simulink model "RT_ueb3_3a"  (R2013a)
settings: Solver=ode45  StartTime=0.0  StopTime=10.0  RelTol=1e-3
settings Model: BufferReuse=off  Creator=mainster  LastModifiedBy=mainster
settings OptimizationCC: InlineParams=on  BufferReuse=off
settings DebuggingCC: InitInArrayFormatMsg=none

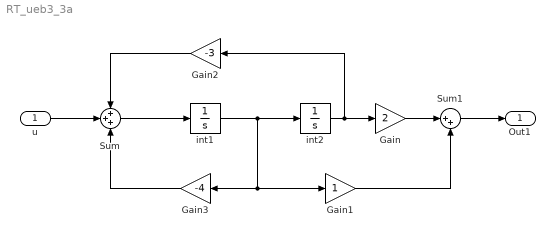
== system RT_ueb3_3a ==
  u : Inport
  Gain : Gain  Gain=2
  Gain1 : Gain
  Gain2 : Gain  Gain=-3
  Gain3 : Gain  Gain=-4
  Sum : Sum  Inputs=+++
  Sum1 : Sum  Inputs=|++
  int1 : Integrator
  int2 : Integrator
  Out1 : Outport
  wires:
  u/1 -> Sum/2
  Sum/1 -> int1/1
  int1/1 -> Gain3/1, Gain1/1, int2/1
  Gain2/1 -> Sum/1
  int2/1 -> Gain/1, Gain2/1
  Gain/1 -> Sum1/1
  Gain1/1 -> Sum1/2
  Sum1/1 -> Out1/1
  Gain3/1 -> Sum/3
